simulink model "DSimulator_robot3GDL"  (Simulink 10.0)
settings: Solver=ode1  StartTime=0  StopTime=30  FixedStep=0.004  RelTol=1e-3  EnableMultiTasking=on
undefined symbols (not defined in the file or in its folder): Dinamic_ur10_3DOF, SimpleRobotPlotROS, Tau, TrajGen
libraries: simulink x3
settings Model: Creator=E. Dean  LastModifiedBy=dominik
settings DataIOCC: LimitDataPoints=on  SignalLoggingSaveFormat=ModelDataLogs
settings OptimizationCC: ExpressionDepthLimit=2147483647
settings DebuggingCC: SolverPrmCheckMsg=warning  FcnCallInpInsideContextMsg=warning  AllowSymbolicDim=off  StateNameClashWarn=warning
settings GRTTargetCC: GeneratePreprocessorConditionals=Disable all
settings ConfigComp: CovExternalEMLEnable=off  CovSFcnEnable=off

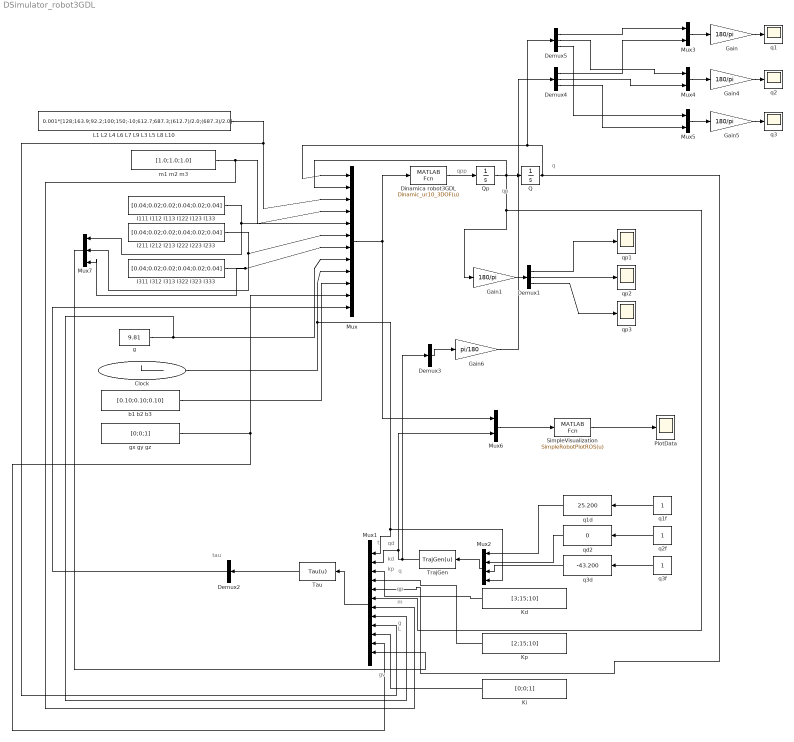
== system DSimulator_robot3GDL ==
  note: gv
  note: qd
  note: q
  note: qp
  note: qpp
  note: tau
  note: t
  note: L
  note: g
  note: m
  note: kp
  note: kd
  note: qp
  note: q
  Clock : Clock
  Demux1 : Demux  Outputs=3
  Demux2 : Demux  Outputs=1
  Demux3 : Demux  Outputs=1
  Demux4 : Demux  Outputs=3
  Demux5 : Demux  Outputs=3
  Dinamica robot3GDL : MATLABFcn  MATLABFcn=Dinamic_ur10_3DOF(u)  OutputDimensions=3
  Gain{,1,4..5} (4 alike) : Gain  Gain=180/pi
  Gain6 : Gain  Gain=pi/180
  I111 I112 I113 I122 I123 I133 : Constant  Value=[0.04;0.02;0.02;0.04;0.02;0.04]
  I211 I212 I213 I222 I223 I233 : Constant  Value=[0.04;0.02;0.02;0.04;0.02;0.04]
  I311 I312 I313 I322 I323 I333 : Constant  Value=[0.04;0.02;0.02;0.04;0.02;0.04]
  "Kd " : Constant  Value=[3;15;10]
  Ki : Constant  Value=[0;0;1]
  Kp : Constant  Value=[2;15;10]
  "L1 L2 L4 L6 L7 L9 L3 L5 L8 L10 " : Constant  Value=0.001*[128;163.9;92.2;100;150;-10;612.7;687.3;(612.7)/2.0;(687.3)/2.0]
  Mux : Mux  Inputs=12
  Mux1 : Mux  Inputs=12
  Mux2 : Mux
  Mux{3..6} (4 alike) : Mux  Inputs=2
  Mux7 : Mux  Inputs=3
  PlotData : Scope
  Q : Integrator  InitialCondition=[0;0;0]
  Qp : Integrator  InitialCondition=[0;0;0]
  SimpleVisualization : MATLABFcn  MATLABFcn=SimpleRobotPlotROS(u)  OutputDimensions=3
  "Tau " : MATLABFcn  MATLABFcn=Tau(u)  OutputDimensions=9
  TrajGen : MATLABFcn  MATLABFcn=TrajGen(u)  OutputDimensions=9
  "b1 b2 b3 " : Constant  Value=[0.10;0.10;0.10]
  g : Constant  Value=9.81
  gx gy gz : Constant  Value=[0;0;1]
  "m1 m2 m3 " : Constant  Value=[1.0;1.0;1.0]
  q1 : Scope
  q1d : simulink/Math Operations/Slider Gain  gain=25.200  low=-180  high=180
  q1f : Constant
  q2 : Scope
  q2f : Constant
  q3 : Scope
  q3d : simulink/Math Operations/Slider Gain  gain=-43.200  low=-180  high=180
  q3f : Constant
  qd2 : simulink/Math Operations/Slider Gain  gain=0  low=-180  high=180
  qp1 : Scope
  qp2 : Scope
  qp3 : Scope
  wires:
  Dinamica robot3GDL/1 -> Qp/1
  Gain/1 -> q1/1
  Gain1/1 -> Demux1/1
  Demux1/1 -> qp1/1
  Demux1/2 -> qp2/1
  Demux1/3 -> qp3/1
  I111 I112 I113 I122 I123 I133/1 -> Mux7/1, Mux/5
  I311 I312 I313 I322 I323 I333/1 -> Mux7/3, Mux/7
  "b1 b2 b3 "/1 -> Mux/10
  Mux/1 -> Mux6/1, Dinamica robot3GDL/1
  Mux1/1 -> "Tau "/1
  TrajGen/1 -> Demux3/1, Mux6/2, Mux1/2
  q1f/1 -> q1d/1
  q2f/1 -> qd2/1
  q3f/1 -> q3d/1
  Mux2/1 -> TrajGen/1
  q1d/1 -> Mux2/1
  qd2/1 -> Mux2/2
  q3d/1 -> Mux2/3
  "Kd "/1 -> Mux1/3
  Kp/1 -> Mux1/4
  Q/1 -> Demux5/1, Mux/1, Mux1/5
  Qp/1 -> Q/1, Mux1/6, Gain1/1, Mux/2
  "Tau "/1 -> Demux2/1
  "m1 m2 m3 "/1 -> Mux1/7, Mux/4
  g/1 -> Mux1/8, Mux/8
  "L1 L2 L4 L6 L7 L9 L3 L5 L8 L10 "/1 -> Mux1/9, Mux/3
  Clock/1 -> Mux2/4, Mux1/1, Mux/9
  Ki/1 -> Mux1/10
  Demux3/1 -> Gain6/1
  Demux4/1 -> Mux3/2
  Mux3/1 -> Gain/1
  Gain4/1 -> q2/1
  Mux4/1 -> Gain4/1
  Gain5/1 -> q3/1
  Mux5/1 -> Gain5/1
  Demux5/1 -> Mux3/1
  Demux5/2 -> Mux4/1
  Gain6/1 -> Demux4/1
  Mux6/1 -> SimpleVisualization/1
  Demux2/1 -> Mux/12
  gx gy gz/1 -> Mux1/11, Mux/11
  Demux5/3 -> Mux5/1
  Demux4/2 -> Mux4/2
  Demux4/3 -> Mux5/2
  I211 I212 I213 I222 I223 I233/1 -> Mux7/2, Mux/6
  Mux7/1 -> Mux1/12
  SimpleVisualization/1 -> PlotData/1
